simulink model "Final_Version"  (R2021b)
settings: Solver=VariableStepAuto  StartTime=0.0  StopTime=380  RelTol=1e-3
values from neighbouring files (symbols this model uses):
  a = a/2    (= 0.1)    [DOF6Script.m]
  b = b/2    (= -0.25)    [DOF6Script.m]
  c = c/2    (= 1000)    [DOF6Script.m]
  d = d/2    (= 1000)    [DOF6Script.m]
  K = 1.11    [DOF6Script.m]
undefined symbols (not defined in the file or in its folder): Continuous, Time
libraries: simulink x29, cstblocks x13, mpclib x3, ctrlSharedLib x1
settings Model: Creator=alela  LastModifiedBy=alela
settings DebuggingCC: UnderSpecifiedDimensionMsg=error

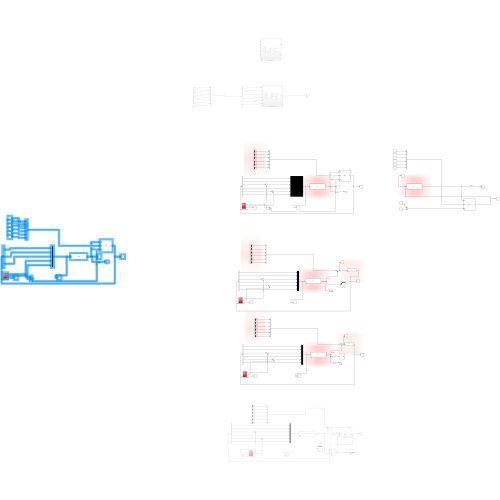
[thumbnail: Simulink's stored preview of the top-level diagram]
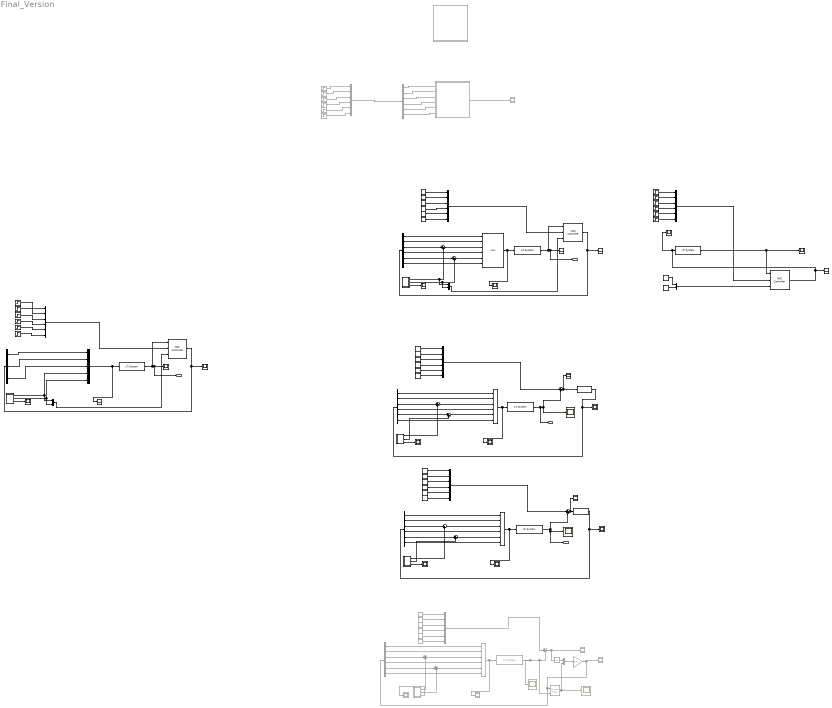
== system Final_Version ==
  Constant : Constant  Value=0
  Constant1 : Constant  Value=0
  Demux : Demux  Commented=on  Outputs=6
  Demux1 : Demux  Outputs=6
  Demux2 : Demux  Outputs=6
  Demux3 : Demux  Outputs=6
  Demux4 : Demux  Commented=on  Outputs=6
  Demux5 : Demux  Outputs=3
  Gain : Gain  Commented=on  Gain=K  Multiplication=Matrix(K*u)
  Integrator : Integrator  Commented=on
  Kalman Filter : ctrlSharedLib/Kalman Filter  Commented=on  TimeDomain=Continuous-Time  UseCurrentEstimator=on  ModelSource=LTI State-Space Variable  ModelSourceVariable=linsys1  A=0.95  B=1  C=1  D=0  NumberOfStates=1  NumberOfInputs=1  NumberOfOutputs=1  InitialEstimateSource=Dialog  X0=0  P0=10  UseK=off  UseGH=off  NumberOfProcessNoiseInputs=1  G=1  TimeInvariantG=on  H=0  TimeInvariantH=on  Q=0.05  TimeInvariantQ=on  R=1  TimeInvariantR=on  N=0  TimeInvariantN=on  AddInputPort=on  AddEnablePort=off  OutputEstimatedY=off  OutputP=off  Ts=-1
  LTI System{,1,3,6} (4 alike) : cstblocks/LTI System  sys=linsys1  IC=[]
  LTI System2 : cstblocks/LTI System  sys=K_mix  IC=[]
  LTI System4 : cstblocks/LTI System  sys=K_PID  IC=[]
  LTI System5 : cstblocks/LTI System  Commented=on  sys=linsys1  IC=[]
  LTI System7 : cstblocks/LTI System  sys=linsys2  IC=[]
  MPC Controller1 : mpclib/MPC Controller  SCDEnableBlockLinearizationSpecification=on  mpcobj=mpc1  is_multiple=0  enable_value=0  return_u0=off  updateMPCinCallerWorkspace=on  md_inport=on  mv_inport=off  uref_inport=off  return_cost=off  return_mvseq=off  return_qpstatus=off  return_xseq=off  return_state=off  return_ovseq=off  state_inport=off  umin_inport=off  umax_inport=off  ymin_inport=off  ymax_inport=off  cc_inport=off  ywt_inport=off  uwt_inport=off  duwt_inport=off  rhoeps_inport=off  pm_inport=off  MaximumP=10  HorizonChoice=FixedHorizon  n_ts=0.1  n_p=15  n_mv=6  n_md=2  n_ud=0  n_mo=6  n_uo=0  BlockDataType=double  SampleTimeInherited=off  switch_inport=off
  MPC Controller2 : mpclib/MPC Controller  SCDEnableBlockLinearizationSpecification=on  mpcobj=mpc1  is_multiple=0  enable_value=0  return_u0=off  updateMPCinCallerWorkspace=on  md_inport=on  mv_inport=off  uref_inport=off  return_cost=off  return_mvseq=off  return_qpstatus=off  return_xseq=off  return_state=off  return_ovseq=off  state_inport=off  umin_inport=off  umax_inport=off  ymin_inport=off  ymax_inport=off  cc_inport=off  ywt_inport=off  uwt_inport=off  duwt_inport=off  rhoeps_inport=off  pm_inport=off  MaximumP=10  HorizonChoice=FixedHorizon  n_ts=0.1  n_p=15  n_mv=6  n_md=2  n_ud=0  n_mo=6  n_uo=0  BlockDataType=double  SampleTimeInherited=off  switch_inport=off
  MPC Controller3 : mpclib/MPC Controller  SCDEnableBlockLinearizationSpecification=on  is_multiple=0  enable_value=0  return_u0=off  updateMPCinCallerWorkspace=on  md_inport=on  mv_inport=off  uref_inport=off  return_cost=off  return_mvseq=off  return_qpstatus=off  return_xseq=off  return_state=off  return_ovseq=off  state_inport=off  umin_inport=off  umax_inport=off  ymin_inport=off  ymax_inport=off  cc_inport=off  ywt_inport=off  uwt_inport=off  duwt_inport=off  rhoeps_inport=off  pm_inport=off  MaximumP=10  HorizonChoice=FixedHorizon  n_ts=0.1  n_p=15  n_mv=3  n_md=2  n_ud=0  n_mo=6  n_uo=0  BlockDataType=double  SampleTimeInherited=off  switch_inport=off
  Mux : Mux  Commented=on  Inputs=6
  Mux{1..4,6..7,12,14} (8 alike) : Mux  Inputs=6
  Mux10 : Mux  Commented=on  Inputs=2
  Mux11 : Mux  Inputs=5
  Mux13 : Mux  Inputs=2
  Mux15 : Mux  Inputs=2
  Mux5 : Mux  Inputs=2
  Mux8 : Mux  Commented=on  Inputs=6
  Mux9 : Mux  Commented=on  Inputs=6
  Repeating Sequence Stair : simulink/Sources/Repeating Sequence Stair  OutValues=x_trajectory  tsamp=sample_time  OutMin=[]  OutMax=[]  OutDataTypeStr=double  OutputDataTypeScalingMode=double  OutDataType=fixdt(0,8)  ConRadixGroup=Best Precision: Vector-wise  OutScaling=2^-12
  Repeating Sequence Stair1 : simulink/Sources/Repeating Sequence Stair  OutValues=z_trajectory  tsamp=sample_time  OutMin=[]  OutMax=[]  OutDataTypeStr=double  OutputDataTypeScalingMode=double  OutDataType=fixdt(0,8)  ConRadixGroup=Best Precision: Vector-wise  OutScaling=2^-12
  Repeating Sequence Stair10 : simulink/Sources/Repeating Sequence Stair  OutValues=pich_trajectory  tsamp=sample_time  OutMin=[]  OutMax=[]  OutDataTypeStr=double  OutputDataTypeScalingMode=double  OutDataType=fixdt(0,8)  ConRadixGroup=Best Precision: Vector-wise  OutScaling=2^-12
  Repeating Sequence Stair11 : simulink/Sources/Repeating Sequence Stair  OutValues=yaw_trajectory  tsamp=sample_time  OutMin=[]  OutMax=[]  OutDataTypeStr=double  OutputDataTypeScalingMode=double  OutDataType=fixdt(0,8)  ConRadixGroup=Best Precision: Vector-wise  OutScaling=2^-12
  Repeating Sequence Stair12 : simulink/Sources/Repeating Sequence Stair  OutValues=pich_trajectory  tsamp=sample_time  OutMin=[]  OutMax=[]  OutDataTypeStr=double  OutputDataTypeScalingMode=double  OutDataType=fixdt(0,8)  ConRadixGroup=Best Precision: Vector-wise  OutScaling=2^-12
  Repeating Sequence Stair13 : simulink/Sources/Repeating Sequence Stair  OutValues=yaw_trajectory  tsamp=sample_time  OutMin=[]  OutMax=[]  OutDataTypeStr=double  OutputDataTypeScalingMode=double  OutDataType=fixdt(0,8)  ConRadixGroup=Best Precision: Vector-wise  OutScaling=2^-12
  Repeating Sequence Stair14 : simulink/Sources/Repeating Sequence Stair  OutValues=x_trajectory  tsamp=sample_time  OutMin=[]  OutMax=[]  OutDataTypeStr=double  OutputDataTypeScalingMode=double  OutDataType=fixdt(0,8)  ConRadixGroup=Best Precision: Vector-wise  OutScaling=2^-12
  Repeating Sequence Stair15 : simulink/Sources/Repeating Sequence Stair  OutValues=z_trajectory  tsamp=sample_time  OutMin=[]  OutMax=[]  OutDataTypeStr=double  OutputDataTypeScalingMode=double  OutDataType=fixdt(0,8)  ConRadixGroup=Best Precision: Vector-wise  OutScaling=2^-12
  Repeating Sequence Stair16 : simulink/Sources/Repeating Sequence Stair  OutValues=y_trajectory  tsamp=sample_time  OutMin=[]  OutMax=[]  OutDataTypeStr=double  OutputDataTypeScalingMode=double  OutDataType=fixdt(0,8)  ConRadixGroup=Best Precision: Vector-wise  OutScaling=2^-12
  Repeating Sequence Stair17 : simulink/Sources/Repeating Sequence Stair  OutValues=roll_trajectory  tsamp=sample_time  OutMin=[]  OutMax=[]  OutDataTypeStr=double  OutputDataTypeScalingMode=double  OutDataType=fixdt(0,8)  ConRadixGroup=Best Precision: Vector-wise  OutScaling=2^-12
  Repeating Sequence Stair18 : simulink/Sources/Repeating Sequence Stair  Commented=on  OutValues=pich_trajectory  tsamp=sample_time  OutMin=[]  OutMax=[]  OutDataTypeStr=double  OutputDataTypeScalingMode=double  OutDataType=fixdt(0,8)  ConRadixGroup=Best Precision: Vector-wise  OutScaling=2^-12
  Repeating Sequence Stair19 : simulink/Sources/Repeating Sequence Stair  Commented=on  OutValues=yaw_trajectory  tsamp=sample_time  OutMin=[]  OutMax=[]  OutDataTypeStr=double  OutputDataTypeScalingMode=double  OutDataType=fixdt(0,8)  ConRadixGroup=Best Precision: Vector-wise  OutScaling=2^-12
  Repeating Sequence Stair2 : simulink/Sources/Repeating Sequence Stair  OutValues=y_trajectory  tsamp=sample_time  OutMin=[]  OutMax=[]  OutDataTypeStr=double  OutputDataTypeScalingMode=double  OutDataType=fixdt(0,8)  ConRadixGroup=Best Precision: Vector-wise  OutScaling=2^-12
  Repeating Sequence Stair20 : simulink/Sources/Repeating Sequence Stair  Commented=on  OutValues=x_trajectory  tsamp=sample_time  OutMin=[]  OutMax=[]  OutDataTypeStr=double  OutputDataTypeScalingMode=double  OutDataType=fixdt(0,8)  ConRadixGroup=Best Precision: Vector-wise  OutScaling=2^-12
  Repeating Sequence Stair21 : simulink/Sources/Repeating Sequence Stair  Commented=on  OutValues=z_trajectory  tsamp=sample_time  OutMin=[]  OutMax=[]  OutDataTypeStr=double  OutputDataTypeScalingMode=double  OutDataType=fixdt(0,8)  ConRadixGroup=Best Precision: Vector-wise  OutScaling=2^-12
  Repeating Sequence Stair22 : simulink/Sources/Repeating Sequence Stair  Commented=on  OutValues=y_trajectory  tsamp=sample_time  OutMin=[]  OutMax=[]  OutDataTypeStr=double  OutputDataTypeScalingMode=double  OutDataType=fixdt(0,8)  ConRadixGroup=Best Precision: Vector-wise  OutScaling=2^-12
  Repeating Sequence Stair23 : simulink/Sources/Repeating Sequence Stair  Commented=on  OutValues=roll_trajectory  tsamp=sample_time  OutMin=[]  OutMax=[]  OutDataTypeStr=double  OutputDataTypeScalingMode=double  OutDataType=fixdt(0,8)  ConRadixGroup=Best Precision: Vector-wise  OutScaling=2^-12
  Repeating Sequence Stair3 : simulink/Sources/Repeating Sequence Stair  OutValues=roll_trajectory  tsamp=sample_time  OutMin=[]  OutMax=[]  OutDataTypeStr=double  OutputDataTypeScalingMode=double  OutDataType=fixdt(0,8)  ConRadixGroup=Best Precision: Vector-wise  OutScaling=2^-12
  Repeating Sequence Stair4 : simulink/Sources/Repeating Sequence Stair  OutValues=pich_trajectory  tsamp=sample_time  OutMin=[]  OutMax=[]  OutDataTypeStr=double  OutputDataTypeScalingMode=double  OutDataType=fixdt(0,8)  ConRadixGroup=Best Precision: Vector-wise  OutScaling=2^-12
  Repeating Sequence Stair5 : simulink/Sources/Repeating Sequence Stair  OutValues=yaw_trajectory  tsamp=sample_time  OutMin=[]  OutMax=[]  OutDataTypeStr=double  OutputDataTypeScalingMode=double  OutDataType=fixdt(0,8)  ConRadixGroup=Best Precision: Vector-wise  OutScaling=2^-12
  Repeating Sequence Stair6 : simulink/Sources/Repeating Sequence Stair  OutValues=x_trajectory  tsamp=sample_time  OutMin=[]  OutMax=[]  OutDataTypeStr=double  OutputDataTypeScalingMode=double  OutDataType=fixdt(0,8)  ConRadixGroup=Best Precision: Vector-wise  OutScaling=2^-12
  Repeating Sequence Stair7 : simulink/Sources/Repeating Sequence Stair  OutValues=z_trajectory  tsamp=sample_time  OutMin=[]  OutMax=[]  OutDataTypeStr=double  OutputDataTypeScalingMode=double  OutDataType=fixdt(0,8)  ConRadixGroup=Best Precision: Vector-wise  OutScaling=2^-12
  Repeating Sequence Stair8 : simulink/Sources/Repeating Sequence Stair  OutValues=y_trajectory  tsamp=sample_time  OutMin=[]  OutMax=[]  OutDataTypeStr=double  OutputDataTypeScalingMode=double  OutDataType=fixdt(0,8)  ConRadixGroup=Best Precision: Vector-wise  OutScaling=2^-12
  Repeating Sequence Stair9 : simulink/Sources/Repeating Sequence Stair  OutValues=roll_trajectory  tsamp=sample_time  OutMin=[]  OutMax=[]  OutDataTypeStr=double  OutputDataTypeScalingMode=double  OutDataType=fixdt(0,8)  ConRadixGroup=Best Precision: Vector-wise  OutScaling=2^-12
  Scope{,15..20} (7 alike) : Scope  Commented=on
  Scope{1..14,21..27} (21 alike) : Scope
  Step{,1..5,9,13..17} (12 alike) : Step  SampleTime=0
  Step{6..8,10..12} (6 alike) : Step  Commented=on  SampleTime=0
  Submarine : Subsystem  Commented=on
  Submarine1 : Subsystem  Commented=on
  Sum{,1..3,5..6} (6 alike) : Sum  Inputs=|++
  Sum10 : Sum  Commented=on  Inputs=|+-
  Sum4 : Sum  Inputs=|+-
  Sum7 : Sum  Inputs=|+-
  Sum8 : Sum  Commented=on  Inputs=|++
  Sum9 : Sum  Commented=on  Inputs=|++
  Wave Disturbance1 : Subsystem
  Wave Disturbance2 : Subsystem
  Wave Disturbance3 : Subsystem
  Wave Disturbance4 : Subsystem  Commented=on
  Wave Disturbance5 : Subsystem
  Out1 : Outport
  out_Hinf : Outport  Port=2
  out_PID : Outport  Port=3
  Out2 : Outport  Port=4
  wires:
  Submarine/1(eta) -> Scope/1  "out"
  Demux/6 -> Submarine/6(N)
  Demux/5 -> Submarine/5(M)
  Demux/4 -> Submarine/4(K)
  Demux/3 -> Submarine/3(Z)
  Demux/2 -> Submarine/2(Y)
  Demux/1 -> Submarine/1(X)
  Step12/1 -> Mux/1
  Step11/1 -> Mux/6
  Step7/1 -> Mux/3
  Step6/1 -> Mux/2
  Step8/1 -> Mux/4
  Step10/1 -> Mux/5
  Mux/1 -> Demux/1
  Mux1/1 -> Scope1/1, LTI System/1
  Repeating Sequence Stair4/1 -> Mux2/5
  Repeating Sequence Stair3/1 -> Mux2/4
  Mux2/1 -> MPC Controller1/2
  Repeating Sequence Stair5/1 -> Mux2/6
  LTI System/1 -> Out1/1, Scope2/1, MPC Controller1/1  "out_MPC"
  Demux1/1 -> Mux1/1
  Demux1/4 -> Mux1/4
  Demux1/6 -> Mux1/6
  Demux1/2 -> Mux1/2
  MPC Controller1/1 -> Scope4/1, Demux1/1
  Demux1/3 -> Sum/1
  Demux1/5 -> Sum1/1
  Sum/1 -> Mux1/3
  Sum1/1 -> Mux1/5
  Wave Disturbance1/2(Mw) -> Mux5/2, Sum1/2
  Wave Disturbance1/3(Out3) -> Scope3/1
  Wave Disturbance2/1(Zw) -> Sum2/2
  Sum2/1 -> Mux3/3
  Demux2/6 -> Mux3/6
  LTI System2/1 -> Demux2/1, Scope8/1
  Demux2/1 -> Mux3/1
  Demux2/4 -> Mux3/4
  Demux2/2 -> Mux3/2
  LTI System1/1 -> out_Hinf/1, Sum4/2, Scope6/1  "out_Hinf"
  Sum3/1 -> Mux3/5
  Demux2/3 -> Sum2/1
  Wave Disturbance2/2(Mw) -> Sum3/2
  Demux2/5 -> Sum3/1
  Wave Disturbance2/3(Out3) -> Scope7/1
  Mux4/1 -> Sum4/1
  Sum4/1 -> Scope9/1, LTI System2/1
  Wave Disturbance1/1(Zw) -> Mux5/1, Sum/2
  Mux5/1 -> MPC Controller1/3
  Repeating Sequence Stair/1 -> Mux2/1
  Repeating Sequence Stair2/1 -> Mux2/2
  Repeating Sequence Stair1/1 -> Mux2/3
  Repeating Sequence Stair9/1 -> Mux4/4
  Repeating Sequence Stair11/1 -> Mux4/6
  Repeating Sequence Stair10/1 -> Mux4/5
  Repeating Sequence Stair6/1 -> Mux4/1
  Repeating Sequence Stair7/1 -> Mux4/3
  Repeating Sequence Stair8/1 -> Mux4/2
  Wave Disturbance3/2(Mw) -> Sum6/2
  Repeating Sequence Stair17/1 -> Mux7/4
  Repeating Sequence Stair14/1 -> Mux7/1
  Repeating Sequence Stair15/1 -> Mux7/3
  Repeating Sequence Stair13/1 -> Mux7/6
  Repeating Sequence Stair12/1 -> Mux7/5
  Wave Disturbance3/1(Zw) -> Sum5/2
  LTI System4/1 -> Demux3/1, Scope13/1
  Mux7/1 -> Sum7/1
  Demux3/5 -> Sum6/1
  Sum5/1 -> Mux6/3
  Mux6/1 -> Scope10/1, LTI System3/1
  Demux3/2 -> Mux6/2
  Repeating Sequence Stair16/1 -> Mux7/2
  Wave Disturbance3/3(Out3) -> Scope12/1
  Demux3/3 -> Sum5/1
  Demux3/1 -> Mux6/1
  Demux3/6 -> Mux6/6
  Demux3/4 -> Mux6/4
  Sum6/1 -> Mux6/5
  Sum7/1 -> Scope14/1, LTI System4/1
  LTI System3/1 -> Sum7/2, out_PID/1, Scope11/1  "out_PID"
  Mux3/1 -> Scope5/1, LTI System1/1
  Wave Disturbance4/3(Out3) -> Scope17/1
  Repeating Sequence Stair22/1 -> Mux9/2
  Demux4/2 -> Mux8/2
  Mux8/1 -> Scope15/1, LTI System5/1
  Sum8/1 -> Mux8/3
  Demux4/5 -> Sum9/1
  Mux9/1 -> Sum10/1
  Gain/1 -> Kalman Filter/1, Demux4/1, Scope18/1
  LTI System5/1 -> Kalman Filter/2, Sum10/2, Scope16/1  "out"
  Sum10/1 -> Integrator/1, Scope19/1
  Sum9/1 -> Mux8/5
  Demux4/4 -> Mux8/4
  Demux4/1 -> Mux8/1
  Demux4/6 -> Mux8/6
  Demux4/3 -> Sum8/1
  Repeating Sequence Stair19/1 -> Mux9/6
  Repeating Sequence Stair23/1 -> Mux9/4
  Repeating Sequence Stair18/1 -> Mux9/5
  Wave Disturbance4/2(Mw) -> Sum9/2
  Wave Disturbance4/1(Zw) -> Sum8/2
  Repeating Sequence Stair20/1 -> Mux9/1
  Repeating Sequence Stair21/1 -> Mux9/3
  Integrator/1 -> Mux10/1
  Kalman Filter/1 -> Scope20/1, Mux10/2
  Mux10/1 -> Gain/1
  LTI System6/1 -> Scope22/1, MPC Controller2/1  "out_MPC"
  Mux12/1 -> MPC Controller2/2
  MPC Controller2/1 -> Scope21/1, LTI System6/1, Scope24/1
  Mux13/1 -> MPC Controller2/3
  Step/1 -> Mux12/1
  Step5/1 -> Mux12/6
  Step4/1 -> Mux12/5
  Step3/1 -> Mux12/4
  Step2/1 -> Mux12/3
  Step1/1 -> Mux12/2
  Constant/1 -> Mux13/1
  Constant1/1 -> Mux13/2
  Wave Disturbance5/2(Mw) -> Mux11/5, Mux15/2
  Mux15/1 -> MPC Controller3/3
  Mux11/1 -> Scope23/1, LTI System7/1
  Demux5/2 -> Mux11/2
  MPC Controller3/1 -> Scope27/1, Demux5/1
  Wave Disturbance5/1(Zw) -> Mux11/4, Mux15/1
  Mux14/1 -> MPC Controller3/2
  LTI System7/1 -> Out2/1, Scope25/1, MPC Controller3/1  "out_MPC"
  Wave Disturbance5/3(Out3) -> Scope26/1
  Demux5/1 -> Mux11/1
  Step15/1 -> Mux14/3
  Step16/1 -> Mux14/4
  Step13/1 -> Mux14/1
  Step9/1 -> Mux14/6
  Step17/1 -> Mux14/5
  Demux5/3 -> Mux11/3
  Step14/1 -> Mux14/2

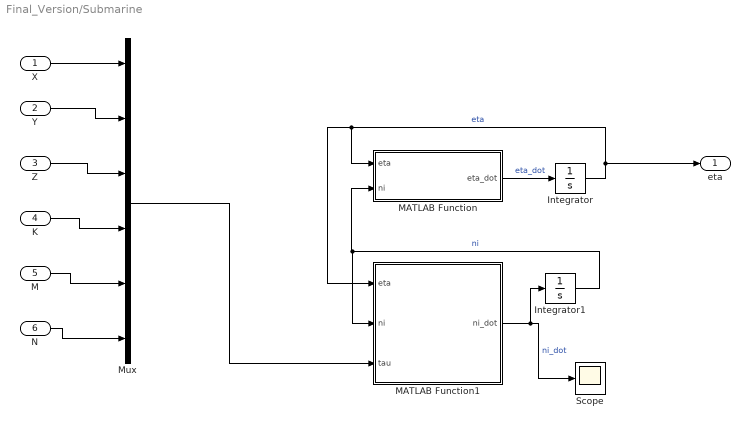
== system Final_Version/Submarine ==
  X : Inport
  Y : Inport  Port=2
  Z : Inport  Port=3
  K : Inport  Port=4
  M : Inport  Port=5
  N : Inport  Port=6
  Integrator : Integrator  ContinuousStateAttributes={'x','y','z','phi','theta','psi'}
  Integrator1 : Integrator  ContinuousStateAttributes={'u','v','w','p','q','r'}
  MATLAB Function : MATLAB Function  TreatAsAtomicUnit=on
  MATLAB Function1 : MATLAB Function  TreatAsAtomicUnit=on
  Mux : Mux  Inputs=6
  Scope : Scope
  eta : Outport
  wires:
  N/1 -> Mux/6
  MATLAB Function/1(eta_dot) -> Integrator/1  "eta_dot"
  Z/1 -> Mux/3
  M/1 -> Mux/5
  Integrator1/1 -> MATLAB Function1/2(ni), MATLAB Function/2(ni)  "ni"
  K/1 -> Mux/4
  Integrator/1 -> eta/1, MATLAB Function1/1(eta), MATLAB Function/1(eta)  "eta"
  MATLAB Function1/1(ni_dot) -> Integrator1/1, Scope/1  "ni_dot"
  Y/1 -> Mux/2
  X/1 -> Mux/1
  Mux/1 -> MATLAB Function1/3(tau)

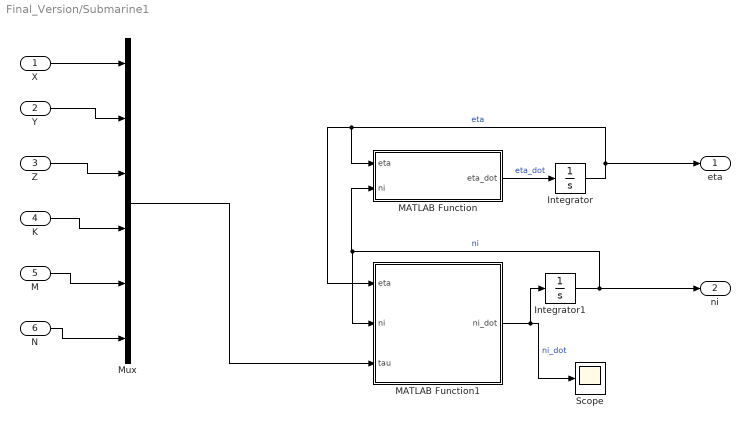
== system Final_Version/Submarine1 ==
  X : Inport
  Y : Inport  Port=2
  Z : Inport  Port=3
  K : Inport  Port=4
  M : Inport  Port=5
  N : Inport  Port=6
  Integrator : Integrator  ContinuousStateAttributes={'x','y','z','phi','theta','psi'}
  Integrator1 : Integrator  ContinuousStateAttributes={'u','v','w','p','q','r'}
  MATLAB Function : MATLAB Function  TreatAsAtomicUnit=on
  MATLAB Function1 : MATLAB Function  TreatAsAtomicUnit=on
  Mux : Mux  Inputs=6
  Scope : Scope
  eta : Outport
  ni : Outport  Port=2
  wires:
  N/1 -> Mux/6
  MATLAB Function/1(eta_dot) -> Integrator/1  "eta_dot"
  Z/1 -> Mux/3
  M/1 -> Mux/5
  Integrator1/1 -> ni/1, MATLAB Function1/2(ni), MATLAB Function/2(ni)  "ni"
  K/1 -> Mux/4
  Integrator/1 -> eta/1, MATLAB Function1/1(eta), MATLAB Function/1(eta)  "eta"
  MATLAB Function1/1(ni_dot) -> Integrator1/1, Scope/1  "ni_dot"
  Y/1 -> Mux/2
  X/1 -> Mux/1
  Mux/1 -> MATLAB Function1/3(tau)

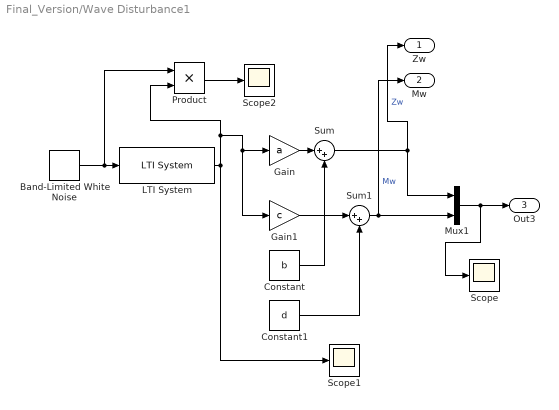
== system Final_Version/Wave Disturbance1 ==
  Band-Limited White Noise : simulink/Sources/Band-Limited White Noise  Cov=[0.1]  Ts=0.01  seed=[23341]
  Constant : Constant  Value=b
  Constant1 : Constant  Value=d
  Gain : Gain  Gain=a
  Gain1 : Gain  Gain=c
  LTI System : cstblocks/LTI System  sys=G4  IC=[]
  Mux1 : Mux  Inputs=2
  Product : Product
  Scope : Scope
  Scope1 : Scope
  Scope2 : Scope
  Sum : Sum  Inputs=|++
  Sum1 : Sum  Inputs=|++
  Zw : Outport
  Mw : Outport  Port=2
  Out3 : Outport  Port=3
  wires:
  Sum/1 -> Zw/1, Mux1/1  "Zw"
  Gain/1 -> Sum/1
  Gain1/1 -> Sum1/1
  Constant/1 -> Sum/2
  Band-Limited White Noise/1 -> Product/1, LTI System/1
  Sum1/1 -> Mux1/2, Mw/1  "Mw"
  Constant1/1 -> Sum1/2
  Mux1/1 -> Scope/1, Out3/1
  LTI System/1 -> Scope1/1, Product/2, Gain1/1, Gain/1
  Product/1 -> Scope2/1

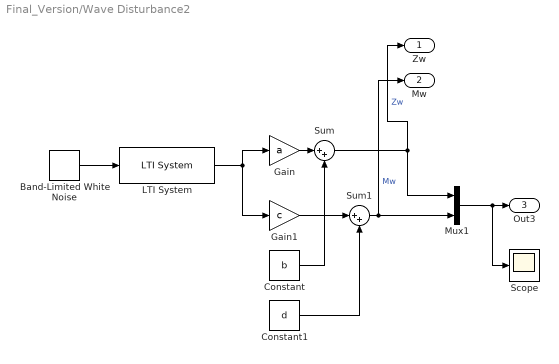
== system Final_Version/Wave Disturbance2 ==
  Band-Limited White Noise : simulink/Sources/Band-Limited White Noise  Cov=[0.1]  Ts=0.01  seed=[23341]
  Constant : Constant  Value=b
  Constant1 : Constant  Value=d
  Gain : Gain  Gain=a
  Gain1 : Gain  Gain=c
  LTI System : cstblocks/LTI System  sys=G4  IC=[]
  Mux1 : Mux  Inputs=2
  Scope : Scope
  Sum : Sum  Inputs=|++
  Sum1 : Sum  Inputs=|++
  Zw : Outport
  Mw : Outport  Port=2
  Out3 : Outport  Port=3
  wires:
  LTI System/1 -> Gain1/1, Gain/1
  Sum/1 -> Zw/1, Mux1/1  "Zw"
  Gain/1 -> Sum/1
  Gain1/1 -> Sum1/1
  Constant/1 -> Sum/2
  Band-Limited White Noise/1 -> LTI System/1
  Sum1/1 -> Mux1/2, Mw/1  "Mw"
  Constant1/1 -> Sum1/2
  Mux1/1 -> Scope/1, Out3/1

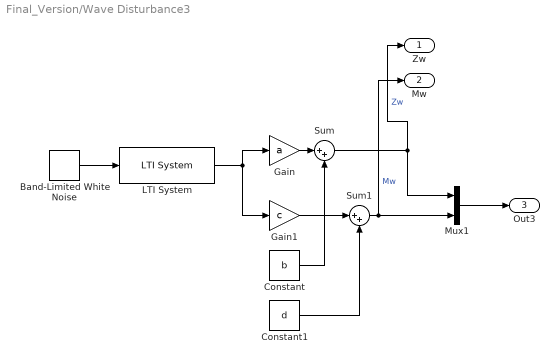
== system Final_Version/Wave Disturbance3 ==
  Band-Limited White Noise : simulink/Sources/Band-Limited White Noise  Cov=[0.1]  Ts=0.01  seed=[23341]
  Constant : Constant  Value=b
  Constant1 : Constant  Value=d
  Gain : Gain  Gain=a
  Gain1 : Gain  Gain=c
  LTI System : cstblocks/LTI System  sys=G4  IC=[]
  Mux1 : Mux  Inputs=2
  Sum : Sum  Inputs=|++
  Sum1 : Sum  Inputs=|++
  Zw : Outport
  Mw : Outport  Port=2
  Out3 : Outport  Port=3
  wires:
  LTI System/1 -> Gain1/1, Gain/1
  Sum/1 -> Zw/1, Mux1/1  "Zw"
  Gain/1 -> Sum/1
  Gain1/1 -> Sum1/1
  Constant/1 -> Sum/2
  Band-Limited White Noise/1 -> LTI System/1
  Sum1/1 -> Mux1/2, Mw/1  "Mw"
  Constant1/1 -> Sum1/2
  Mux1/1 -> Out3/1

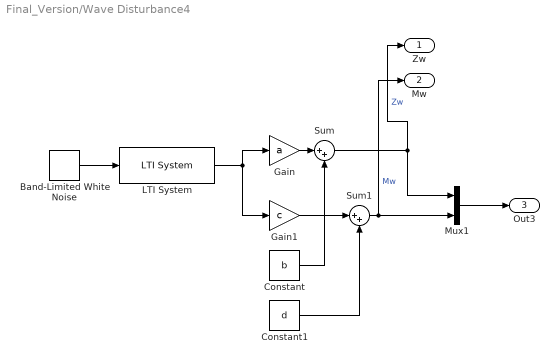
== system Final_Version/Wave Disturbance4 ==
  Band-Limited White Noise : simulink/Sources/Band-Limited White Noise  Cov=[0.1]  Ts=0.01  seed=[23341]
  Constant : Constant  Value=b
  Constant1 : Constant  Value=d
  Gain : Gain  Gain=a
  Gain1 : Gain  Gain=c
  LTI System : cstblocks/LTI System  sys=G4  IC=[]
  Mux1 : Mux  Inputs=2
  Sum : Sum  Inputs=|++
  Sum1 : Sum  Inputs=|++
  Zw : Outport
  Mw : Outport  Port=2
  Out3 : Outport  Port=3
  wires:
  LTI System/1 -> Gain1/1, Gain/1
  Sum/1 -> Zw/1, Mux1/1  "Zw"
  Gain/1 -> Sum/1
  Gain1/1 -> Sum1/1
  Constant/1 -> Sum/2
  Band-Limited White Noise/1 -> LTI System/1
  Sum1/1 -> Mux1/2, Mw/1  "Mw"
  Constant1/1 -> Sum1/2
  Mux1/1 -> Out3/1

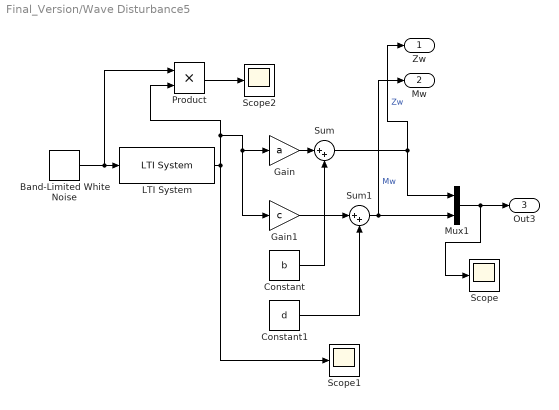
== system Final_Version/Wave Disturbance5 ==
  Band-Limited White Noise : simulink/Sources/Band-Limited White Noise  Cov=[0.1]  Ts=0.01  seed=[23341]
  Constant : Constant  Value=b
  Constant1 : Constant  Value=d
  Gain : Gain  Gain=a
  Gain1 : Gain  Gain=c
  LTI System : cstblocks/LTI System  sys=G4  IC=[]
  Mux1 : Mux  Inputs=2
  Product : Product
  Scope : Scope
  Scope1 : Scope
  Scope2 : Scope
  Sum : Sum  Inputs=|++
  Sum1 : Sum  Inputs=|++
  Zw : Outport
  Mw : Outport  Port=2
  Out3 : Outport  Port=3
  wires:
  Sum/1 -> Zw/1, Mux1/1  "Zw"
  Gain/1 -> Sum/1
  Gain1/1 -> Sum1/1
  Constant/1 -> Sum/2
  Band-Limited White Noise/1 -> Product/1, LTI System/1
  Sum1/1 -> Mux1/2, Mw/1  "Mw"
  Constant1/1 -> Sum1/2
  Mux1/1 -> Scope/1, Out3/1
  LTI System/1 -> Scope1/1, Product/2, Gain1/1, Gain/1
  Product/1 -> Scope2/1

== matlab function Final_Version/Submarine/MATLAB Function1 ==
  data: eta input size=6; ni_dot output size=6; ni input size=6; tau input size=6

function ni_dot = ni_dot_fcn(eta,ni,tau)
    
    m = 5454.54; %(kg)
    g = 9.81; %(m/s^2)
    Izx = -13.58; %(Nms^2)
    Ixz = -13.58; %(Nms^2)
    Ix = 2038; %(Nms^2)
    Iz = 13587; %(Nms^2)
    Iy = 13587; %(Nm^2)
    zg = 0.061; %(m)
    rho = 1000; %(kg/m^3)
    r = 5.3; %(m)   
    Delta = m/rho; %(m^3)
    xg = 0;
    xb = 0;
    zb = 0;
    Xq = -1.5*10^(-2);
    Xu = 5.3*10^(-2);   Zu=-6.8*10^(-2);    Kv=3.1*10^(-3);   Mu=-2.6*10^(-2);  Nv = -7.4*10^(-3);
    Xw = 1.7*10^(-3);   Zw=-3.0*10^(-1);    Kp=-1.1*10^(-2);  Mv=-2.6*10^(-2);  Np = -8.4*10^(-4);
    Yv = -10*10^(-1);   Zq=-1.4*10^(-1);    Kr=-8.4*10^(-4);  Mq=-1.6*10^(-3);  Nr = -1.6*10^(-2);
    Yp = 3.0*10^(-3);                                         Mw= 1.0*10^(-1);
    Yr = 3.0*10^(-2);
    
    Xu_dot = -7.6*10^(-3); Yv_dot=-5.5*10^(-2);   Zu_dot=-3.0*10^(-2);  Kv_dot = 1.2*10^(-4);  Mu_dot = -6.8*10^(-3);  Nv_dot = 1.2*10^(-3);
    Xw_dot = 1.7*10^(-3);  Yp_dot=1.2*10^(-4);    Zw_dot=-2.4*10^(-1);  Kp_dot = -1.0*10^(-3); Mw_dot = -6.8*10^(-3);  Np_dot = -3.4*10^(-5);
    Xq_dot = 2.5*10^(-2);  Yr_dot= 1.2*10^(-3);   Zq_dot=-6.8*10^(-3);  Kr_dot = -3.4*10^(-5); Mq_dot = -1.7*10^(-2);  Nr_dot = -3.4*10^(-3);

    % Take eta signal
    x = eta(1);
    y = eta(2);
    z = eta(3);
    phi = eta(4);
    theta = eta(5);
    psi = eta(6);

    % Take v signal
    u = ni(1);
    v = ni(2);
    w = ni(3);
    p = ni(4);
    q = ni(5);
    r = ni(6);

    % Build M matrix

    M = [m-Xu_dot       0        -Xw_dot         0        m*zg-Xq_dot       0;
        0             m-Yv_dot       0       -m*zg-Yp_dot       0       m*xg-Yr_dot;
      -Xw_dot            0        m-Zw_dot       0        -m*xg-Zq_dot       0;
        0           -m*zg-Yp_dot     0       Ix-Kp_dot          0       -Izx-Kr_dot;
    m*zg-Xq_dot           0     -m*xg-Zq_dot     0          Iy-Mq_dot        0;
        0            m*xg-Yr_dot     0       -Izx-Kr_dot        0        Iz-Nr_dot];

    %Corioli Centripetal matrix coefficintes

    a1 = Xu_dot*u + Xw_dot*w + Xq_dot*q;
    a2 = Yv_dot*v + Yp_dot*p + Yr_dot*r;
    a3 = Zu_dot*u + Zw_dot*w + Zq_dot*r;
    b1 = Kv_dot*v + Kp_dot*p + Kr_dot*r;
    b2 = Mu_dot*u + Mw_dot*w + Mq_dot*q;
    b3 = Nv_dot*v + Np_dot*p + Nr_dot*r;

    Ca = [0  0  0  0  -a3  a2;
          0  0  0  a3  0  -a1;
          0  0  0  -a2 a1  0;
          0 -a3 a2  0  -b3  b2;
          a3  0  -a1 b3  0  -b1;
          -a2  a1  0  -b2  b1  0];

    C_rb=[0 -m*r m*q m*zg*r -m*xg*q -m*xg*r;
          m*r 0 -m*p 0 m*(zg*r+xg*p) 0;
          -m*q m*p 0 -m*zg*p -m*zg*q m*xg*p;
          -m*zg*r 0 m*zg*p 0 -Ixz*p+Iz*r -Iy*q;
          m*xg*q -m*(zg*r+xg*p) m*zg*q Ixz*p-Iz*r 0 -Ixz*r+Ix*p;
          m*xg*r 0 -m*xg*p Iy*q Ixz*r-Ix*p 0];

    D=-[Xu 0 Xw 0 Xq 0;
        0 Yv 0 Yp 0 Yr;
        Zu 0 Zw 0 Zq 0;
        0 Kv 0 Kp 0 Kr;
        Mu 0 Mw 0 Mq 0;
        0 Nv 0 Np 0 Nr];
    
    W=m*g;
    B=rho*g*Delta;
    Aut=(W-B);
    G=[Aut*sin(theta);
       -Aut*sin(phi)*cos(theta);
       -Aut*cos(phi)*cos(theta);
       (zg*W-zb*B)*sin(phi)*cos(theta);
       (zg*W-zb*B)*sin(theta)+(xg*W-xb*B)*cos(theta)*cos(phi);
       -(xg*W-xb*B)*cos(theta)*sin(phi)];

%ni_dot=M/(tau-(Ca+C_rb)*ni-G-D*ni);
ni_dot=inv(M)*(tau-(Ca+C_rb)*ni-G-D*ni);

== matlab function Final_Version/Submarine/MATLAB Function ==
  data: eta input size=6; eta_dot output size=6; ni input

function eta_dot = eta_dot_fcn(eta,ni)
    
    % Take eta signal
    x = eta(1);
    y = eta(2);
    z = eta(3);
    phi = eta(4);
    theta = eta(5);
    psi = eta(6);

    % Take v signal
    u = ni(1);
    v = ni(2);
    w = ni(3);
    p = ni(4);
    q = ni(5);
    r = ni(6);

    %Build Rotation matrix
    
    R = [cos(psi)*cos(theta)  -sin(psi)*cos(phi)+cos(psi)*sin(theta)*sin(phi)  sin(psi)*sin(phi)+cos(psi)*cos(theta)*sin(theta);
        sin(psi)*cos(theta)              cos(psi)*cos(phi)+sin(phi)*sin(psi)     -cos(psi)*sin(phi) + sin(theta)*sin(psi)*cos(phi);
        -sin(theta)                              cos(theta)*sin(phi)                            cos(theta)*cos(phi)       ];

    % Build coordinate transformation matrix
    
    T = [1      sin(phi)*tan(theta)          cos(phi)*tan(theta);
        0       cos(phi)                    -sin(phi);
        0       sin(phi)/cos(theta)           cos(phi)/cos(theta)];

    zero = zeros(3);

    J = [R      zero;
        zero      T];
    
eta_dot = J*ni;

== matlab function Final_Version/Submarine1/MATLAB Function ==
  data: eta input size=6; eta_dot output size=6; ni input

function eta_dot = eta_dot_fcn(eta,ni)
    
    % Take eta signal
    x = eta(1);
    y = eta(2);
    z = eta(3);
    phi = eta(4);
    theta = eta(5);
    psi = eta(6);

    % Take v signal
    u = ni(1);
    v = ni(2);
    w = ni(3);
    p = ni(4);
    q = ni(5);
    r = ni(6);

    %Build Rotation matrix
    
    R = [cos(psi)*cos(theta)  -sin(psi)*cos(phi)+cos(psi)*sin(theta)*sin(phi)  sin(psi)*sin(phi)+cos(psi)*cos(theta)*sin(theta);
        sin(psi)*cos(theta)              cos(psi)*cos(phi)+sin(phi)*sin(psi)     -cos(psi)*sin(phi) + sin(theta)*sin(psi)*cos(phi);
        -sin(theta)                              cos(theta)*sin(phi)                            cos(theta)*cos(phi)       ];

    % Build coordinate transformation matrix
    
    T = [1      sin(phi)*tan(theta)          cos(phi)*tan(theta);
        0       cos(phi)                    -sin(phi);
        0       sin(phi)/cos(theta)           cos(phi)/cos(theta)];

    zero = zeros(3);

    J = [R      zero;
        zero      T];
    
eta_dot = J*ni;

== matlab function Final_Version/Submarine1/MATLAB Function1 ==
  data: eta input size=6; ni_dot output size=6; ni input size=6; tau input size=6

function ni_dot = ni_dot_fcn(eta,ni,tau)
    
    m = 5454.54; %(kg)
    g = 9.81; %(m/s^2)
    Izx = -13.58; %(Nms^2)
    Ixz = -13.58; %(Nms^2)
    Ix = 2038; %(Nms^2)
    Iz = 13587; %(Nms^2)
    Iy = 13587; %(Nm^2)
    zg = 0.061; %(m)
    rho = 1000; %(kg/m^3)
    r = 5.3; %(m)   
    Delta = m/rho; %(m^3)
    xg = 0;
    xb = 0;
    zb = 0;
    Xq = -1.5*10^(-2);
    Xu = 5.3*10^(-2);   Zu=-6.8*10^(-2);    Kv=3.1*10^(-3);   Mu=-2.6*10^(-2);  Nv = -7.4*10^(-3);
    Xw = 1.7*10^(-3);   Zw=-3.0*10^(-1);    Kp=-1.1*10^(-2);  Mv=-2.6*10^(-2);  Np = -8.4*10^(-4);
    Yv = -10*10^(-1);   Zq=-1.4*10^(-1);    Kr=-8.4*10^(-4);  Mq=-1.6*10^(-3);  Nr = -1.6*10^(-2);
    Yp = 3.0*10^(-3);                                         Mw= 1.0*10^(-1);
    Yr = 3.0*10^(-2);
    
    Xu_dot = -7.6*10^(-3); Yv_dot=-5.5*10^(-2);   Zu_dot=-3.0*10^(-2);  Kv_dot = 1.2*10^(-4);  Mu_dot = -6.8*10^(-3);  Nv_dot = 1.2*10^(-3);
    Xw_dot = 1.7*10^(-3);  Yp_dot=1.2*10^(-4);    Zw_dot=-2.4*10^(-1);  Kp_dot = -1.0*10^(-3); Mw_dot = -6.8*10^(-3);  Np_dot = -3.4*10^(-5);
    Xq_dot = 2.5*10^(-2);  Yr_dot= 1.2*10^(-3);   Zq_dot=-6.8*10^(-3);  Kr_dot = -3.4*10^(-5); Mq_dot = -1.7*10^(-2);  Nr_dot = -3.4*10^(-3);

    % Take eta signal
    x = eta(1);
    y = eta(2);
    z = eta(3);
    phi = eta(4);
    theta = eta(5);
    psi = eta(6);

    % Take v signal
    u = ni(1);
    v = ni(2);
    w = ni(3);
    p = ni(4);
    q = ni(5);
    r = ni(6);

    % Build M matrix

    M = [m-Xu_dot       0        -Xw_dot         0        m*zg-Xq_dot       0;
        0             m-Yv_dot       0       -m*zg-Yp_dot       0       m*xg-Yr_dot;
      -Xw_dot            0        m-Zw_dot       0        -m*xg-Zq_dot       0;
        0           -m*zg-Yp_dot     0       Ix-Kp_dot          0       -Izx-Kr_dot;
    m*zg-Xq_dot           0     -m*xg-Zq_dot     0          Iy-Mq_dot        0;
        0            m*xg-Yr_dot     0       -Izx-Kr_dot        0        Iz-Nr_dot];

    %Corioli Centripetal matrix coefficintes

    a1 = Xu_dot*u + Xw_dot*w + Xq_dot*q;
    a2 = Yv_dot*v + Yp_dot*p + Yr_dot*r;
    a3 = Zu_dot*u + Zw_dot*w + Zq_dot*r;
    b1 = Kv_dot*v + Kp_dot*p + Kr_dot*r;
    b2 = Mu_dot*u + Mw_dot*w + Mq_dot*q;
    b3 = Nv_dot*v + Np_dot*p + Nr_dot*r;

    Ca = [0  0  0  0  -a3  a2;
          0  0  0  a3  0  -a1;
          0  0  0  -a2 a1  0;
          0 -a3 a2  0  -b3  b2;
          a3  0  -a1 b3  0  -b1;
          -a2  a1  0  -b2  b1  0];

    C_rb=[0 -m*r m*q m*zg*r -m*xg*q -m*xg*r;
          m*r 0 -m*p 0 m*(zg*r+xg*p) 0;
          -m*q m*p 0 -m*zg*p -m*zg*q m*xg*p;
          -m*zg*r 0 m*zg*p 0 -Ixz*p+Iz*r -Iy*q;
          m*xg*q -m*(zg*r+xg*p) m*zg*q Ixz*p-Iz*r 0 -Ixz*r+Ix*p;
          m*xg*r 0 -m*xg*p Iy*q Ixz*r-Ix*p 0];

    D=-[Xu 0 Xw 0 Xq 0;
        0 Yv 0 Yp 0 Yr;
        Zu 0 Zw 0 Zq 0;
        0 Kv 0 Kp 0 Kr;
        Mu 0 Mw 0 Mq 0;
        0 Nv 0 Np 0 Nr];
    
    W=m*g;
    B=rho*g*Delta;
    Aut=(W-B);
    G=[Aut*sin(theta);
       -Aut*sin(phi)*cos(theta);
       -Aut*cos(phi)*cos(theta);
       (zg*W-zb*B)*sin(phi)*cos(theta);
       (zg*W-zb*B)*sin(theta)+(xg*W-xb*B)*cos(theta)*cos(phi);
       -(xg*W-xb*B)*cos(theta)*sin(phi)];

%ni_dot=M/(tau-(Ca+C_rb)*ni-G-D*ni);
ni_dot=inv(M)*(tau-(Ca+C_rb)*ni-G-D*ni);
